simulink model "sh_controller"  (R2021b)
settings: Solver=FixedStepAuto  StartTime=0.0  StopTime=t_stop  FixedStep=1e-3  RelTol=1e-3
undefined symbols (not defined in the file or in its folder): DiscIntNeverNeededParam
settings Model: Creator=Luca  LastModifiedBy=albertogagliardi
settings DataIOCC: SignalLogging=off  DSMLogging=off  ReturnWorkspaceOutputs=off

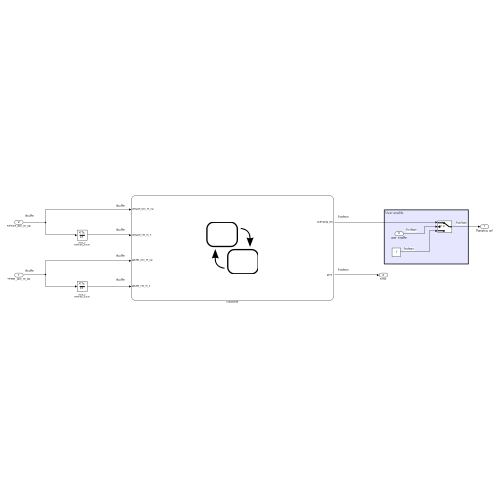
[thumbnail: Simulink's stored preview of the top-level diagram]
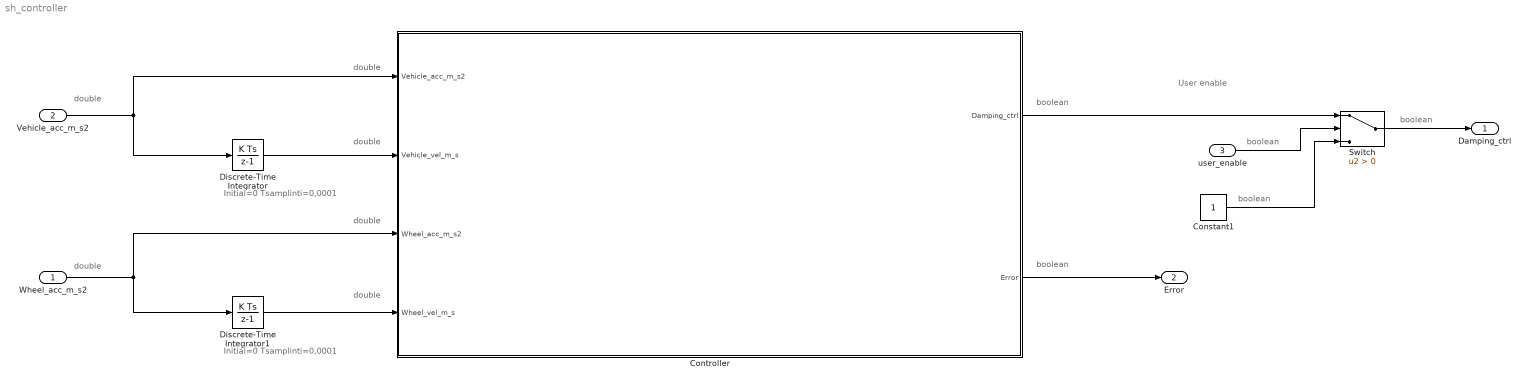
== system sh_controller ==
  note: Initial=0
      | Tsamplinti=0,0001
  note: boolean
  note: boolean
  note: boolean
  note: boolean
  note: boolean
  note: double
  note: double
  note: double
  note: double
  note: Initial=0
      | Tsamplinti=0,0001
  note: double
  note: double
  note: User enable
  Wheel_acc_m_s2 : Inport
  Vehicle_acc_m_s2 : Inport  Port=2
  user_enable : Inport  Port=3  OutDataTypeStr=boolean
  Constant1 : Constant  OutDataTypeStr=boolean
  Controller : Stateflow chart  TreatAsAtomicUnit=on
  Discrete-Time Integrator : DiscreteIntegrator  SampleTime=-1  ICPrevOutput=DiscIntNeverNeededParam  ICPrevScaledInput=DiscIntNeverNeededParam
  Discrete-Time Integrator1 : DiscreteIntegrator  SampleTime=-1  ICPrevOutput=DiscIntNeverNeededParam  ICPrevScaledInput=DiscIntNeverNeededParam
  Switch : Switch  Criteria=u2 > Threshold
  Damping_ctrl : Outport
  Error : Outport  Port=2
  wires:
  Controller/1(Damping_ctrl) -> Switch/1
  Controller/2(Error) -> Error/1
  Discrete-Time Integrator/1 -> Controller/2(Vehicle_vel_m_s)
  Vehicle_acc_m_s2/1 -> Controller/1(Vehicle_acc_m_s2), Discrete-Time Integrator/1
  Discrete-Time Integrator1/1 -> Controller/4(Wheel_vel_m_s)
  Wheel_acc_m_s2/1 -> Controller/3(Wheel_acc_m_s2), Discrete-Time Integrator1/1
  Switch/1 -> Damping_ctrl/1
  user_enable/1 -> Switch/2
  Constant1/1 -> Switch/3

== stateflow chart sh_controller/Controller ==
  state Controller_logic [parallel]
    settings: executionOrder=1
    state Normal_working
      state High_damping
        en:
        Damping_ctrl = 1;
      state Low_damping
        en:
        Damping_ctrl = 0;
      (default) -> High_damping
      High_damping -> Low_damping : [(Vehicle_vel_m_s-Wheel_vel_m_s)*Vehicle_vel_m_s<0]
      Low_damping -> High_damping : [(Vehicle_vel_m_s-Wheel_vel_m_s)*Vehicle_vel_m_s>=0]
    state Emergency_working
      en:
      Damping_ctrl = 1;
    (default) -> Normal_working
    Normal_working -> Emergency_working : [Error~=0]
  state Vehicle_check [parallel]
    settings: executionOrder=3
    state OK_vehicle
      en:
      Vehicle_acc_prev_prev = Vehicle_acc_prev;
      Vehicle_acc_prev = Vehicle_acc_m_s2;
    state Error_vehicle
      en:
      Error = 2;
    (junction 126) -> (junction 128) : [Vehicle_acc_prev>Vehicle_acc_prev_prev-1e-5 && Vehicle_acc_prev<Vehicle_acc_prev_prev+1e-5]
    OK_vehicle -> (junction 126) [order 3]
    (junction 128) -> OK_vehicle : {
        | counter_vehicle=counter_vehicle+1;
        | }
    (default) -> OK_vehicle
    OK_vehicle -> Error_vehicle [order 1] : [counter_vehicle>=20]
    OK_vehicle -> (junction 113) [order 2]
    (junction 114) -> OK_vehicle : {
        | counter_vehicle=0;
        | }
    (junction 113) -> (junction 114) : [Vehicle_acc_prev<=Vehicle_acc_prev_prev-1e-5 || Vehicle_acc_prev>=Vehicle_acc_prev_prev+1e-5]
  state Wheel_check [parallel]
    settings: executionOrder=2
    state OK_wheel
      en:
      Wheel_acc_prev_prev = Wheel_acc_prev;
      Wheel_acc_prev = Wheel_acc_m_s2;
    state Error_wheel
      en:
      Error = 1;
    (junction 133) -> (junction 135) : [Wheel_acc_prev>Wheel_acc_prev_prev-1e-5 && Wheel_acc_prev<Wheel_acc_prev_prev+1e-5]
    OK_wheel -> (junction 133) [order 3]
    (junction 135) -> OK_wheel : {
        | counter_wheel=counter_wheel+1;
        | }
    (default) -> OK_wheel
    OK_wheel -> Error_wheel [order 1] : [counter_wheel>=20]
    OK_wheel -> (junction 100) [order 2]
    (junction 101) -> OK_wheel : {
        | counter_wheel=0;
        | }
    (junction 100) -> (junction 101) : [Wheel_acc_prev<=Wheel_acc_prev_prev-1e-5 || Wheel_acc_prev>=Wheel_acc_prev_prev+1e-5]
  data: Vehicle_acc_prev local double =-1; Vehicle_acc_prev_prev local double =-2; counter_vehicle local int8 =0; Wheel_acc_prev local double =-1; Wheel_acc_prev_prev local double =-2; counter_wheel local int8 =0; Vehicle_acc_m_s2 input double; Vehicle_vel_m_s input double; Wheel_acc_m_s2 input double; Wheel_vel_m_s input double; Damping_ctrl output boolean; Error output int8 =0
